simulink model "pha_0_9"  (R2023a)
settings: Solver=VariableStepAuto  StartTime=0.0  StopTime=100  RelTol=1e-3
libraries: fl_lib x55, SimscapeFluids_lib x25, nesl_utility x15, slpidlib x2, simulink x1
(part 2 of 2)

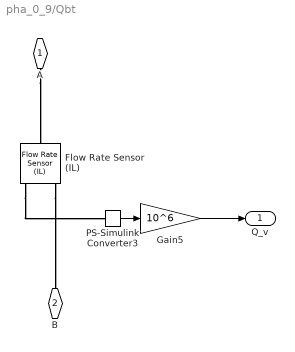
== system pha_0_9/Qbt ==
  Flow Rate Sensor (IL) : fl_lib/Isothermal Liquid/Sensors/Flow Rate Sensor (IL)  sensor_type=foundation.enum.mass_volumetric_sensor.mass_volumetric
      settings: InternalSimscapePortConfiguration="{\"Bottom\":[],\"Left\":[{\"id\":\"A\",\"label\":\"A\",\"type\":\"foundation.isothermal_liquid.isothermal_liquid\"}],\"Right\":[{\"id\":\"B\",\"label\":\"B\",\"type\":\"foundation.isothermal_liquid.isothermal_liquid\"},{\"id\":\"M\",\"label\":\"M\",\"type\":\"output\"},{\"id\":\"V\",\"label\":\"V\",\"type\":\"output\"}],\"Top\":[]}"
  Gain5 : Gain  Gain=10^6
  PS-Simulink Converter3 : nesl_utility/PS-Simulink Converter  PhysicalDomain=network_engine_domain  SubClassName=ps_output  LeftPortType=input  RightPortType=output  PseudoPeriodic=off  Frequencies=[]  VectorFormat=inherit  Unit=inherit  AffineConversion=off
  A : PMIOPort  Side=Left
  B : PMIOPort  Port=2  Side=Right
  Q_v : Outport
  wires:
  PS-Simulink Converter3/1 -> Gain5/1
  Gain5/1 -> Q_v/1
  connections:
  Flow Rate Sensor (IL)/RConn1 -- B/RConn1
  A/RConn1 -- Flow Rate Sensor (IL)/LConn1
  Flow Rate Sensor (IL)/RConn3 -- PS-Simulink Converter3/LConn1

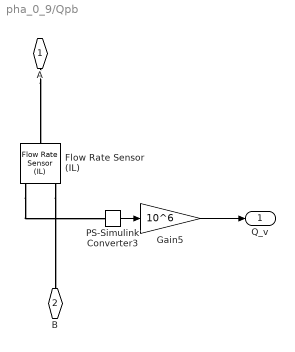
== system pha_0_9/Qpb ==
  Flow Rate Sensor (IL) : fl_lib/Isothermal Liquid/Sensors/Flow Rate Sensor (IL)  sensor_type=foundation.enum.mass_volumetric_sensor.mass_volumetric
      settings: InternalSimscapePortConfiguration="{\"Bottom\":[],\"Left\":[{\"id\":\"A\",\"label\":\"A\",\"type\":\"foundation.isothermal_liquid.isothermal_liquid\"}],\"Right\":[{\"id\":\"B\",\"label\":\"B\",\"type\":\"foundation.isothermal_liquid.isothermal_liquid\"},{\"id\":\"M\",\"label\":\"M\",\"type\":\"output\"},{\"id\":\"V\",\"label\":\"V\",\"type\":\"output\"}],\"Top\":[]}"
  Gain5 : Gain  Gain=10^6
  PS-Simulink Converter3 : nesl_utility/PS-Simulink Converter  PhysicalDomain=network_engine_domain  SubClassName=ps_output  LeftPortType=input  RightPortType=output  PseudoPeriodic=off  Frequencies=[]  VectorFormat=inherit  Unit=inherit  AffineConversion=off
  A : PMIOPort  Side=Left
  B : PMIOPort  Port=2  Side=Right
  Q_v : Outport
  wires:
  PS-Simulink Converter3/1 -> Gain5/1
  Gain5/1 -> Q_v/1
  connections:
  Flow Rate Sensor (IL)/RConn1 -- B/RConn1
  A/RConn1 -- Flow Rate Sensor (IL)/LConn1
  Flow Rate Sensor (IL)/RConn3 -- PS-Simulink Converter3/LConn1

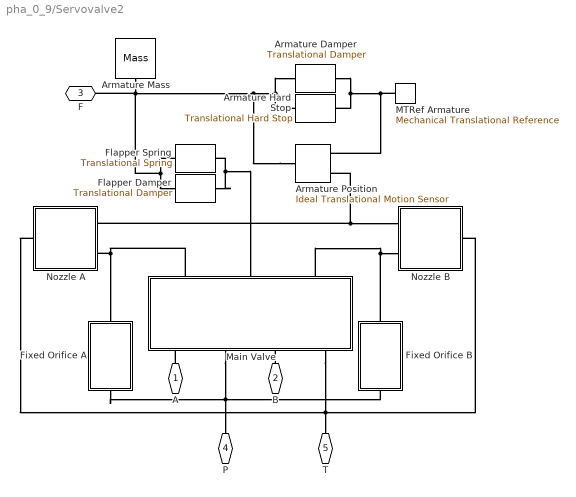
== system pha_0_9/Servovalve2 ==
  Armature Mass : fl_lib/Mechanical/Translational Elements/Mass  Tag=Factory Generic  mass=0.035 kg  num_ports=foundation.enum.numPorts2.one  v_specify=on  v_priority=High  v=0 m/s  v_nominal_specify=off  v_nominal_unit=m/s  v_nominal_value=1  f_specify=off  f_priority=High  f=0 N  f_nominal_specify=off  f_nominal_unit=N  f_nominal_value=1
  Armature Position : fl_lib/Mechanical/Mechanical Sensors/Ideal Translational Motion Sensor  Tag=Factory Generic  reference=foundation.enum.MeasurementReference.difference  acceleration_port=false  velocity_port=true  position_port=true  offset=0 m
  Armature Damper : fl_lib/Mechanical/Translational Elements/Translational Damper  Tag=Factory Generic  D=12.5 N/(m/s)  v_specify=off  v_priority=High  v=0 m/s  v_nominal_specify=off  v_nominal_unit=m/s  v_nominal_value=1  f_specify=off  f_priority=High  f=0 N  f_nominal_specify=off  f_nominal_unit=N  f_nominal_value=1
  Armature Hard Stop : fl_lib/Mechanical/Translational Elements/Translational Hard Stop  Tag=Factory Generic  upper_bnd=0.5 mm  lower_bnd=-0.5 mm  model=3  stiff_up=1e+06 N/m  stiff_low=1e+06 N/m  D_up=150 N/(m/s)  D_low=150 N/(m/s)  transition=0.1 mm  coeff_rest=0.7  v_tol=0.001 m/s  f_tol=0.001 N  x_specify=on  x_priority=High  x=0 m  x_nominal_specify=off  x_nominal_unit=m  x_nominal_value=1  v_specify=off  v_priority=High  v=0 m/s  v_nominal_specify=off  v_nominal_unit=m/s  v_nominal_value=1  f_specify=off  f_priority=High  f=0 N  f_nominal_specify=off  f_nominal_unit=N  f_nominal_value=1  M_specify=off  M_priority=None  M=0
  Fixed Orifice A : Subsystem
  Fixed Orifice B : Subsystem
  Flapper Damper : fl_lib/Mechanical/Translational Elements/Translational Damper  Tag=Factory Generic  D=51 N/(m/s)  v_specify=off  v_priority=High  v=0 m/s  v_nominal_specify=off  v_nominal_unit=m/s  v_nominal_value=1  f_specify=off  f_priority=High  f=0 N  f_nominal_specify=off  f_nominal_unit=N  f_nominal_value=1
  Flapper Spring : fl_lib/Mechanical/Translational Elements/Translational Spring  Tag=Factory Generic  spr_rate=1200 N/m  v_specify=off  v_priority=High  v=0 m/s  v_nominal_specify=off  v_nominal_unit=m/s  v_nominal_value=1  f_specify=off  f_priority=High  f=0 N  f_nominal_specify=off  f_nominal_unit=N  f_nominal_value=1  x_specify=on  x_priority=High  x=0 m  x_nominal_specify=off  x_nominal_unit=m  x_nominal_value=1
  MTRef Armature : fl_lib/Mechanical/Translational Elements/Mechanical Translational Reference  Tag=Factory Generic
  Main Valve : Subsystem  Tag=PublishSubsystem
  Nozzle A : Subsystem
  Nozzle B : Subsystem
  A : PMIOPort  Side=Left
  B : PMIOPort  Port=2  Side=Left
  F : PMIOPort  Port=3  Side=Right
  P : PMIOPort  Port=4  Side=Right
  T : PMIOPort  Port=5  Side=Right
  connections:
  Main Valve/RConn2 -- Fixed Orifice B/LConn1 -- Fixed Orifice A/LConn1 -- P/RConn1
  Armature Position/LConn1 -- Flapper Spring/LConn1 -- Flapper Damper/LConn1 -- F/RConn1 -- Armature Mass/LConn1 -- Armature Damper/LConn1 -- Armature Hard Stop/LConn1
  A/RConn1 -- Main Valve/RConn1
  B/RConn1 -- Main Valve/RConn3
  Flapper Damper/RConn1 -- Flapper Spring/RConn1 -- Main Valve/LConn2
  MTRef Armature/LConn1 -- Armature Position/RConn1 -- Armature Damper/RConn1 -- Armature Hard Stop/RConn1
  Main Valve/LConn1 -- Nozzle A/LConn2 -- Fixed Orifice A/RConn1
  Armature Position/RConn3 -- Nozzle B/LConn1 -- Nozzle A/LConn1
  Fixed Orifice B/RConn1 -- Main Valve/LConn3 -- Nozzle B/LConn2
  Nozzle A/RConn1 -- Nozzle B/RConn1 -- T/RConn1 -- Main Valve/RConn4

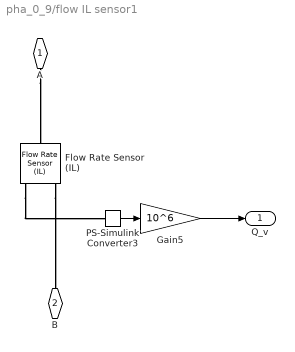
== system pha_0_9/flow IL sensor1 ==
  Flow Rate Sensor (IL) : fl_lib/Isothermal Liquid/Sensors/Flow Rate Sensor (IL)  sensor_type=foundation.enum.mass_volumetric_sensor.mass_volumetric
      settings: InternalSimscapePortConfiguration="{\"Bottom\":[],\"Left\":[{\"id\":\"A\",\"label\":\"A\",\"type\":\"foundation.isothermal_liquid.isothermal_liquid\"}],\"Right\":[{\"id\":\"B\",\"label\":\"B\",\"type\":\"foundation.isothermal_liquid.isothermal_liquid\"},{\"id\":\"M\",\"label\":\"M\",\"type\":\"output\"},{\"id\":\"V\",\"label\":\"V\",\"type\":\"output\"}],\"Top\":[]}"
  Gain5 : Gain  Gain=10^6
  PS-Simulink Converter3 : nesl_utility/PS-Simulink Converter  PhysicalDomain=network_engine_domain  SubClassName=ps_output  LeftPortType=input  RightPortType=output  PseudoPeriodic=off  Frequencies=[]  VectorFormat=inherit  Unit=inherit  AffineConversion=off
  A : PMIOPort  Side=Left
  B : PMIOPort  Port=2  Side=Right
  Q_v : Outport
  wires:
  PS-Simulink Converter3/1 -> Gain5/1
  Gain5/1 -> Q_v/1
  connections:
  Flow Rate Sensor (IL)/RConn1 -- B/RConn1
  A/RConn1 -- Flow Rate Sensor (IL)/LConn1
  Flow Rate Sensor (IL)/RConn3 -- PS-Simulink Converter3/LConn1

== system pha_0_9/flow sensor1 ==
  Flow Rate Sensor (TL)3 : fl_lib/Thermal Liquid/Sensors/Flow Rate Sensor (TL)  mass_flow_measure=true  volumetric_flow_measure=true  energy_flow_measure=true
      settings: InternalSimscapePortConfiguration="{\"Bottom\":[{\"id\":\"PHI\",\"label\":\"φ\",\"type\":\"output\"}],\"Left\":[{\"id\":\"A\",\"label\":\"A\",\"type\":\"foundation.thermal_liquid.thermal_liquid\"}],\"Right\":[{\"id\":\"B\",\"label\":\"B\",\"type\":\"foundation.thermal_liquid.thermal_liquid\"},{\"id\":\"M\",\"label\":\"M\",\"type\":\"output\"},{\"id\":\"V\",\"label\":\"V\",\"type\":\"output\"}],\"Top\":[]}"
  Gain5 : Gain  Gain=10^6
  PS-Simulink Converter3 : nesl_utility/PS-Simulink Converter  PhysicalDomain=network_engine_domain  SubClassName=ps_output  LeftPortType=input  RightPortType=output  PseudoPeriodic=off  Frequencies=[]  VectorFormat=inherit  Unit=inherit  AffineConversion=off
  A : PMIOPort  Side=Left
  B : PMIOPort  Port=2  Side=Right
  Q_v : Outport
  wires:
  PS-Simulink Converter3/1 -> Gain5/1
  Gain5/1 -> Q_v/1
  connections:
  PS-Simulink Converter3/LConn1 -- Flow Rate Sensor (TL)3/RConn3
  Flow Rate Sensor (TL)3/RConn1 -- B/RConn1
  A/RConn1 -- Flow Rate Sensor (TL)3/LConn1

== system pha_0_9/flow sensor2 ==
  Flow Rate Sensor (TL)3 : fl_lib/Thermal Liquid/Sensors/Flow Rate Sensor (TL)  mass_flow_measure=true  volumetric_flow_measure=true  energy_flow_measure=true
      settings: InternalSimscapePortConfiguration="{\"Bottom\":[{\"id\":\"PHI\",\"label\":\"φ\",\"type\":\"output\"}],\"Left\":[{\"id\":\"A\",\"label\":\"A\",\"type\":\"foundation.thermal_liquid.thermal_liquid\"}],\"Right\":[{\"id\":\"B\",\"label\":\"B\",\"type\":\"foundation.thermal_liquid.thermal_liquid\"},{\"id\":\"M\",\"label\":\"M\",\"type\":\"output\"},{\"id\":\"V\",\"label\":\"V\",\"type\":\"output\"}],\"Top\":[]}"
  Gain5 : Gain  Gain=10^6
  PS-Simulink Converter3 : nesl_utility/PS-Simulink Converter  PhysicalDomain=network_engine_domain  SubClassName=ps_output  LeftPortType=input  RightPortType=output  PseudoPeriodic=off  Frequencies=[]  VectorFormat=inherit  Unit=inherit  AffineConversion=off
  A : PMIOPort  Side=Left
  B : PMIOPort  Port=2  Side=Right
  Q_v : Outport
  wires:
  PS-Simulink Converter3/1 -> Gain5/1
  Gain5/1 -> Q_v/1
  connections:
  PS-Simulink Converter3/LConn1 -- Flow Rate Sensor (TL)3/RConn3
  Flow Rate Sensor (TL)3/RConn1 -- B/RConn1
  A/RConn1 -- Flow Rate Sensor (TL)3/LConn1

== system pha_0_9/flow sensor3 ==
  Flow Rate Sensor (TL)3 : fl_lib/Thermal Liquid/Sensors/Flow Rate Sensor (TL)  mass_flow_measure=true  volumetric_flow_measure=true  energy_flow_measure=true
      settings: InternalSimscapePortConfiguration="{\"Bottom\":[{\"id\":\"PHI\",\"label\":\"φ\",\"type\":\"output\"}],\"Left\":[{\"id\":\"A\",\"label\":\"A\",\"type\":\"foundation.thermal_liquid.thermal_liquid\"}],\"Right\":[{\"id\":\"B\",\"label\":\"B\",\"type\":\"foundation.thermal_liquid.thermal_liquid\"},{\"id\":\"M\",\"label\":\"M\",\"type\":\"output\"},{\"id\":\"V\",\"label\":\"V\",\"type\":\"output\"}],\"Top\":[]}"
  Gain5 : Gain  Gain=10^6
  PS-Simulink Converter3 : nesl_utility/PS-Simulink Converter  PhysicalDomain=network_engine_domain  SubClassName=ps_output  LeftPortType=input  RightPortType=output  PseudoPeriodic=off  Frequencies=[]  VectorFormat=inherit  Unit=inherit  AffineConversion=off
  A : PMIOPort  Side=Left
  B : PMIOPort  Port=2  Side=Right
  Q_v : Outport
  wires:
  PS-Simulink Converter3/1 -> Gain5/1
  Gain5/1 -> Q_v/1
  connections:
  PS-Simulink Converter3/LConn1 -- Flow Rate Sensor (TL)3/RConn3
  Flow Rate Sensor (TL)3/RConn1 -- B/RConn1
  A/RConn1 -- Flow Rate Sensor (TL)3/LConn1

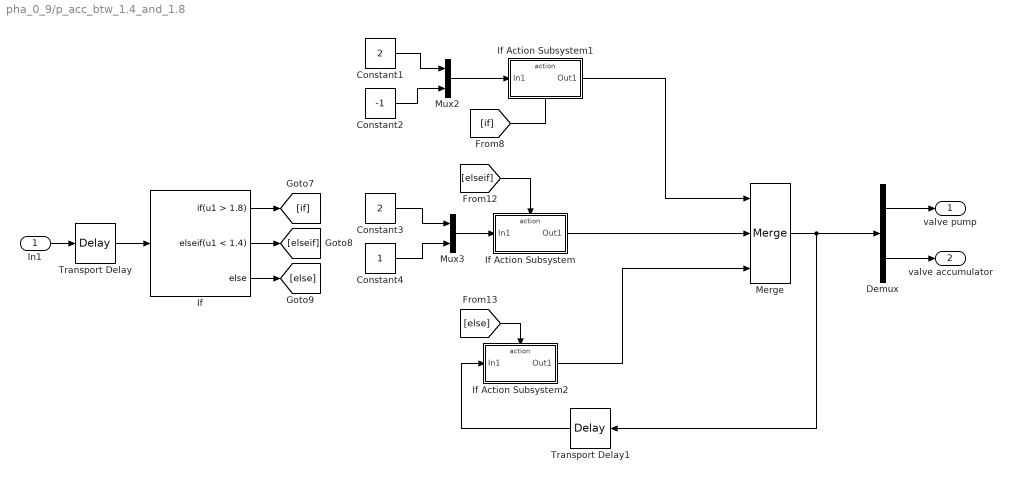
== system pha_0_9/p_acc_btw_1.4_and_1.8 ==
  In1 : Inport
  Constant1 : Constant  Value=2
  Constant2 : Constant  Value=-1
  Constant3 : Constant  Value=2
  Constant4 : Constant
  Demux : Demux  Outputs=2
  If : If  IfExpression=u1 > 1.8  ElseIfExpressions=u1 < 1.4
  If Action Subsystem : Subsystem  TreatAsAtomicUnit=on
  If Action Subsystem1 : Subsystem  TreatAsAtomicUnit=on
  If Action Subsystem2 : Subsystem  TreatAsAtomicUnit=on
  Merge : Merge  Inputs=3
  Mux2 : Mux  Inputs=2
  Mux3 : Mux  Inputs=2
  Transport Delay : TransportDelay  DelayTime=0.001
  Transport Delay1 : TransportDelay  DelayTime=0.001
  valve pump : Outport
  valve accumulator : Outport  Port=2
  wires:
  If/3 -> [else]
  [else] -> If Action Subsystem2/Action
  Merge/1 -> Transport Delay1/1, Demux/1
  Constant3/1 -> Mux3/1
  If/2 -> [elseif]
  Transport Delay1/1 -> If Action Subsystem2/1(In1)
  Constant1/1 -> Mux2/1
  Demux/1 -> valve pump/1
  Constant2/1 -> Mux2/2
  Mux3/1 -> If Action Subsystem/1(In1)
  Constant4/1 -> Mux3/2
  Transport Delay/1 -> If/1
  [elseif] -> If Action Subsystem/Action
  If/1 -> [if]
  Demux/2 -> valve accumulator/1
  In1/1 -> Transport Delay/1
  If Action Subsystem/1(Out1) -> Merge/2
  If Action Subsystem2/1(Out1) -> Merge/3
  If Action Subsystem1/1(Out1) -> Merge/1
  Mux2/1 -> If Action Subsystem1/1(In1)
  [if] -> If Action Subsystem1/Action

== system pha_0_9/pressure sensor ==
  Gain : Gain  Gain=10^(-5)
  PS-Simulink Converter1 : nesl_utility/PS-Simulink Converter  PhysicalDomain=network_engine_domain  SubClassName=ps_output  LeftPortType=input  RightPortType=output  PseudoPeriodic=off  Frequencies=[]  VectorFormat=inherit  Unit=inherit  AffineConversion=off
  Pressure & Temperature Sensor (TL) : fl_lib/Thermal Liquid/Sensors/Pressure & Temperature Sensor (TL)  reference=foundation.enum.MeasurementReference.absolute  pressure=true  pressure_spec=foundation.enum.PressureMeasementSpec.Absolute  temperature=false
      settings: InternalSimscapePortConfiguration="{\"Bottom\":[],\"Left\":[{\"id\":\"A\",\"label\":\"A\",\"type\":\"foundation.thermal_liquid.thermal_liquid\"}],\"Right\":[{\"id\":\"Pa\",\"label\":\"Pa\",\"type\":\"output\"}],\"Top\":[]}"
  A : PMIOPort  Side=Left
  bar : Outport
  wires:
  PS-Simulink Converter1/1 -> Gain/1
  Gain/1 -> bar/1
  connections:
  PS-Simulink Converter1/LConn1 -- Pressure & Temperature Sensor (TL)/RConn1
  Pressure & Temperature Sensor (TL)/LConn1 -- A/RConn1

== system pha_0_9/pressure sensor1 ==
  Gain : Gain  Gain=10^(-5)
  PS-Simulink Converter1 : nesl_utility/PS-Simulink Converter  PhysicalDomain=network_engine_domain  SubClassName=ps_output  LeftPortType=input  RightPortType=output  PseudoPeriodic=off  Frequencies=[]  VectorFormat=inherit  Unit=inherit  AffineConversion=off
  Pressure & Temperature Sensor (TL) : fl_lib/Thermal Liquid/Sensors/Pressure & Temperature Sensor (TL)  reference=foundation.enum.MeasurementReference.absolute  pressure=true  pressure_spec=foundation.enum.PressureMeasementSpec.Absolute  temperature=false
      settings: InternalSimscapePortConfiguration="{\"Bottom\":[],\"Left\":[{\"id\":\"A\",\"label\":\"A\",\"type\":\"foundation.thermal_liquid.thermal_liquid\"}],\"Right\":[{\"id\":\"Pa\",\"label\":\"Pa\",\"type\":\"output\"}],\"Top\":[]}"
  A : PMIOPort  Side=Left
  bar : Outport
  wires:
  PS-Simulink Converter1/1 -> Gain/1
  Gain/1 -> bar/1
  connections:
  PS-Simulink Converter1/LConn1 -- Pressure & Temperature Sensor (TL)/RConn1
  Pressure & Temperature Sensor (TL)/LConn1 -- A/RConn1

== system pha_0_9/pressure sensor2 ==
  Gain : Gain  Gain=10^(-5)
  PS-Simulink Converter1 : nesl_utility/PS-Simulink Converter  PhysicalDomain=network_engine_domain  SubClassName=ps_output  LeftPortType=input  RightPortType=output  PseudoPeriodic=off  Frequencies=[]  VectorFormat=inherit  Unit=inherit  AffineConversion=off
  Pressure & Temperature Sensor (TL) : fl_lib/Thermal Liquid/Sensors/Pressure & Temperature Sensor (TL)  reference=foundation.enum.MeasurementReference.absolute  pressure=true  pressure_spec=foundation.enum.PressureMeasementSpec.Absolute  temperature=false
      settings: InternalSimscapePortConfiguration="{\"Bottom\":[],\"Left\":[{\"id\":\"A\",\"label\":\"A\",\"type\":\"foundation.thermal_liquid.thermal_liquid\"}],\"Right\":[{\"id\":\"Pa\",\"label\":\"Pa\",\"type\":\"output\"}],\"Top\":[]}"
  A : PMIOPort  Side=Left
  bar : Outport
  wires:
  PS-Simulink Converter1/1 -> Gain/1
  Gain/1 -> bar/1
  connections:
  PS-Simulink Converter1/LConn1 -- Pressure & Temperature Sensor (TL)/RConn1
  Pressure & Temperature Sensor (TL)/LConn1 -- A/RConn1

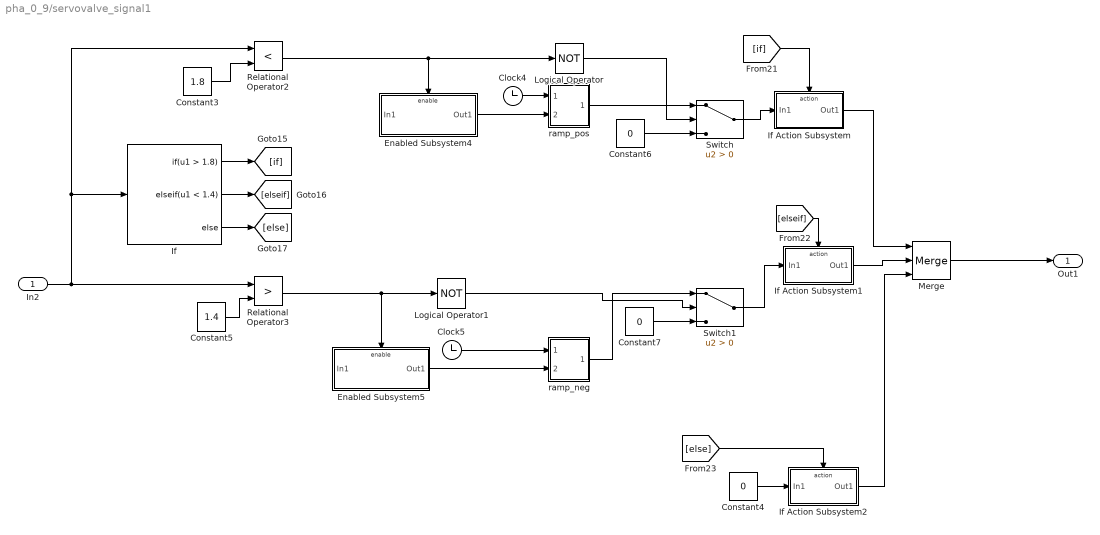
== system pha_0_9/servovalve_signal1 ==
  In2 : Inport
  Clock4 : Clock
  Clock5 : Clock
  Constant3 : Constant  Value=1.8
  Constant4 : Constant  Value=0
  Constant5 : Constant  Value=1.4
  Constant6 : Constant  Value=0
  Constant7 : Constant  Value=0
  Enabled Subsystem4 : Subsystem  TreatAsAtomicUnit=on
  Enabled Subsystem5 : Subsystem  TreatAsAtomicUnit=on
  If : If  IfExpression=u1 > 1.8  ElseIfExpressions=u1 < 1.4
  If Action Subsystem : Subsystem  TreatAsAtomicUnit=on
  If Action Subsystem1 : Subsystem  TreatAsAtomicUnit=on
  If Action Subsystem2 : Subsystem  TreatAsAtomicUnit=on
  Logical Operator : Logic  Operator=NOT  AllPortsSameDT=off  OutDataTypeStr=boolean
  Logical Operator1 : Logic  Operator=NOT  AllPortsSameDT=off  OutDataTypeStr=boolean
  Merge : Merge  Inputs=3
  Relational Operator2 : RelationalOperator  Operator=<  OutDataTypeStr=boolean  RndMeth=Simplest  InputSameDT=off
  Relational Operator3 : RelationalOperator  Operator=>  OutDataTypeStr=boolean  RndMeth=Simplest  InputSameDT=off
  Switch : Switch  Criteria=u2 > Threshold  SaturateOnIntegerOverflow=off  InputSameDT=off
  Switch1 : Switch  Criteria=u2 > Threshold  SaturateOnIntegerOverflow=off  InputSameDT=off
  ramp_neg : Subsystem
  ramp_pos : Subsystem
  Out1 : Outport
  wires:
  Relational Operator2/1 -> Logical Operator/1, Enabled Subsystem4/Enable
  Enabled Subsystem4/1(Out1) -> ramp_pos/2(In2)
  [if] -> If Action Subsystem/Action
  [else] -> If Action Subsystem2/Action
  Relational Operator3/1 -> Logical Operator1/1, Enabled Subsystem5/Enable
  If Action Subsystem1/1(Out1) -> Merge/2
  ramp_neg/1(Out1) -> Switch1/1
  Switch1/1 -> If Action Subsystem1/1(In1)
  In2/1 -> If/1, Relational Operator2/1, Relational Operator3/1
  Merge/1 -> Out1/1
  Logical Operator1/1 -> Switch1/2
  Clock4/1 -> ramp_pos/1(In1)
  Enabled Subsystem5/1(Out1) -> ramp_neg/2(In2)
  Constant4/1 -> If Action Subsystem2/1(In1)
  Switch/1 -> If Action Subsystem/1(In1)
  [elseif] -> If Action Subsystem1/Action
  If Action Subsystem/1(Out1) -> Merge/1
  Constant7/1 -> Switch1/3
  If/2 -> [elseif]
  Constant3/1 -> Relational Operator2/2
  If/1 -> [if]
  Constant6/1 -> Switch/3
  Constant5/1 -> Relational Operator3/2
  Clock5/1 -> ramp_neg/1(In1)
  If Action Subsystem2/1(Out1) -> Merge/3
  Logical Operator/1 -> Switch/2
  If/3 -> [else]
  ramp_pos/1(Out1) -> Switch/1

== system pha_0_9/Servovalve2/Fixed Orifice A ==
  Fixed Orifice A : SimscapeFluids_lib/Isothermal Liquid/Valves & Orifices/Orifices/Orifice (IL)  Tag=Factory Generic  orifice_type=1  constant_orifice_spec=fluids.isothermal_liquid.valves_orifices.orifices.enum.constant_orifice_spec.area  variable_orifice_spec=fluids.isothermal_liquid.valves_orifices.orifices.enum.orifice_spec.linear  orifice_area_constant=2 mm^2  p_diff_TLU_constant=[-4, -3, -2, -1, -.5, 0, .5, 1, 2, 3, 4] MPa  vol_flow_TLU_constant=[-2.44, -2.12, -1.68, -1.22, -.84, 0, .85, 1.21, 1.7, 2.09, 2.41] .* 1e-3 m^3/s  S_min=0 m  del_S=5e-3 m  open_orientation=fluids.isothermal_liquid.valves_orifices.orifices.enum.orifice_orientation.positive  area_max=1e-4 m^2  area_leak=1e-10 m^2  S_TLU=[0, .002, .004, .007, .017] m  orifice_area_TLU=[1e-09, 2.0352e-07, 4.0736e-05, .00011438, .00034356] m^2  area=inf mm^2  Cd=0.7  Re_c=150  smoothing_factor=0.01  pressure_recovery=false  S_vol_flow_TLU=[0, .002, .004, .007, .017] m  p_diff_TLU=[.3, .5, .7] MPa  vol_flow_TLU=1e-3 * [1.7e-05, 2e-05, 2.6e-05; .0035, .0045, .0053; .7, .9, 1.06; 1.96, 2.5, 3; 6, 7.7, 9.13] m^3/s  enable_faults=simscape.enum.onoff.off  fault_action=fluids.enum.FaultOpening.Closed  external_fault=fluids.enum.FaultExternalTrigger.Off  temporal_fault=simscape.enum.onoff.off  fault_time=5 s  report_fault=simscape.enum.assert.action.none
      settings: InternalSimscapePortConfiguration="{\"Bottom\":[],\"Left\":[{\"id\":\"A\",\"label\":\"A\",\"type\":\"foundation.isothermal_liquid.isothermal_liquid\"}],\"Right\":[{\"id\":\"B\",\"label\":\"B\",\"type\":\"foundation.isothermal_liquid.isothermal_liquid\"}],\"Top\":[]}"
  B : PMIOPort  Side=Right
  A : PMIOPort  Port=2  Side=Left
  connections:
  A/RConn1 -- Fixed Orifice A/LConn1
  B/RConn1 -- Fixed Orifice A/RConn1

== system pha_0_9/Servovalve2/Fixed Orifice B ==
  Fixed Orifice B : SimscapeFluids_lib/Isothermal Liquid/Valves & Orifices/Orifices/Orifice (IL)  Tag=Factory Generic  orifice_type=1  constant_orifice_spec=fluids.isothermal_liquid.valves_orifices.orifices.enum.constant_orifice_spec.area  variable_orifice_spec=fluids.isothermal_liquid.valves_orifices.orifices.enum.orifice_spec.linear  orifice_area_constant=2 mm^2  p_diff_TLU_constant=[-4, -3, -2, -1, -.5, 0, .5, 1, 2, 3, 4] MPa  vol_flow_TLU_constant=[-2.44, -2.12, -1.68, -1.22, -.84, 0, .85, 1.21, 1.7, 2.09, 2.41] .* 1e-3 m^3/s  S_min=0 m  del_S=5e-3 m  open_orientation=fluids.isothermal_liquid.valves_orifices.orifices.enum.orifice_orientation.positive  area_max=1e-4 m^2  area_leak=1e-10 m^2  S_TLU=[0, .002, .004, .007, .017] m  orifice_area_TLU=[1e-09, 2.0352e-07, 4.0736e-05, .00011438, .00034356] m^2  area=inf mm^2  Cd=0.7  Re_c=150  smoothing_factor=0.01  pressure_recovery=false  S_vol_flow_TLU=[0, .002, .004, .007, .017] m  p_diff_TLU=[.3, .5, .7] MPa  vol_flow_TLU=1e-3 * [1.7e-05, 2e-05, 2.6e-05; .0035, .0045, .0053; .7, .9, 1.06; 1.96, 2.5, 3; 6, 7.7, 9.13] m^3/s  enable_faults=simscape.enum.onoff.off  fault_action=fluids.enum.FaultOpening.Closed  external_fault=fluids.enum.FaultExternalTrigger.Off  temporal_fault=simscape.enum.onoff.off  fault_time=5 s  report_fault=simscape.enum.assert.action.none
      settings: InternalSimscapePortConfiguration="{\"Bottom\":[],\"Left\":[{\"id\":\"A\",\"label\":\"A\",\"type\":\"foundation.isothermal_liquid.isothermal_liquid\"}],\"Right\":[{\"id\":\"B\",\"label\":\"B\",\"type\":\"foundation.isothermal_liquid.isothermal_liquid\"}],\"Top\":[]}"
  B : PMIOPort  Side=Right
  A : PMIOPort  Port=2  Side=Left
  connections:
  A/RConn1 -- Fixed Orifice B/LConn1
  B/RConn1 -- Fixed Orifice B/RConn1

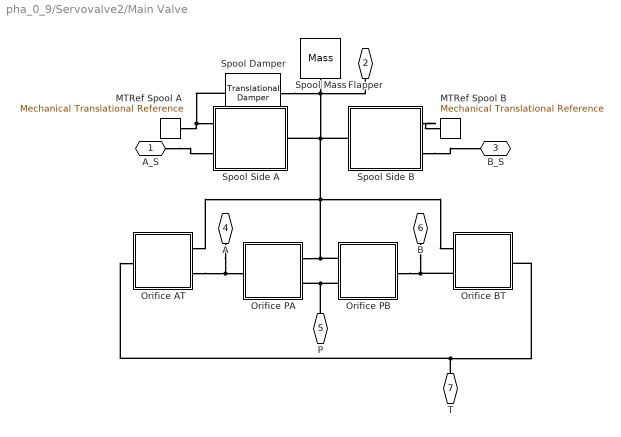
== system pha_0_9/Servovalve2/Main Valve ==
  MTRef Spool A : fl_lib/Mechanical/Translational Elements/Mechanical Translational Reference  Tag=Factory Generic
  MTRef Spool B : fl_lib/Mechanical/Translational Elements/Mechanical Translational Reference  Tag=Factory Generic
  Orifice AT : Subsystem  Tag=PublishSubsystem
  Orifice BT : Subsystem
  Orifice PA : Subsystem
  Orifice PB : Subsystem
  Spool Damper : fl_lib/Mechanical/Translational Elements/Translational Damper  Tag=Factory Generic  D=362 N/(m/s)  v_specify=off  v_priority=High  v=0 m/s  v_nominal_specify=off  v_nominal_unit=m/s  v_nominal_value=1  f_specify=off  f_priority=High  f=0 N  f_nominal_specify=off  f_nominal_unit=N  f_nominal_value=1
  Spool Mass : fl_lib/Mechanical/Translational Elements/Mass  Tag=Factory Generic  mass=0.124 kg  num_ports=foundation.enum.numPorts2.one  v_specify=on  v_priority=High  v=0 m/s  v_nominal_specify=off  v_nominal_unit=m/s  v_nominal_value=1  f_specify=off  f_priority=High  f=0 N  f_nominal_specify=off  f_nominal_unit=N  f_nominal_value=1
  Spool Side A : Subsystem
  Spool Side B : Subsystem
  A_S : PMIOPort  Side=Left
  Flapper : PMIOPort  Port=2  Side=Left
  B_S : PMIOPort  Port=3  Side=Left
  A : PMIOPort  Port=4  Side=Right
  P : PMIOPort  Port=5  Side=Right
  B : PMIOPort  Port=6  Side=Right
  T : PMIOPort  Port=7  Side=Right
  connections:
  A/RConn1 -- Orifice AT/LConn2 -- Orifice PA/RConn1
  P/RConn1 -- Orifice PB/LConn2 -- Orifice PA/LConn2
  Orifice BT/LConn2 -- Orifice PB/RConn1 -- B/RConn1
  T/RConn1 -- Orifice AT/RConn1 -- Orifice BT/RConn1
  MTRef Spool A/LConn1 -- Spool Damper/RConn1 -- Spool Side A/LConn1
  A_S/RConn1 -- Spool Side A/LConn2
  Orifice PA/LConn1 -- Orifice PB/LConn1 -- Orifice BT/LConn1 -- Orifice AT/LConn1 -- Spool Side B/RConn1 -- Spool Side A/RConn1 -- Spool Damper/LConn1 -- Spool Mass/LConn1 -- Flapper/RConn1
  Spool Side B/LConn1 -- MTRef Spool B/LConn1
  Spool Side B/LConn2 -- B_S/RConn1

== system pha_0_9/Servovalve2/Nozzle A ==
  Nozzle A : SimscapeFluids_lib/Isothermal Liquid/Valves & Orifices/Orifices/Orifice (IL)  Tag=Factory Generic  orifice_type=foundation.enum.constant_variable.variable  constant_orifice_spec=fluids.isothermal_liquid.valves_orifices.orifices.enum.constant_orifice_spec.area  variable_orifice_spec=1  orifice_area_constant=1e-3 m^2  p_diff_TLU_constant=[-4, -3, -2, -1, -.5, 0, .5, 1, 2, 3, 4] MPa  vol_flow_TLU_constant=[-2.44, -2.12, -1.68, -1.22, -.84, 0, .85, 1.21, 1.7, 2.09, 2.41] .* 1e-3 m^3/s  S_min=-2.9981e-07 m^2/mm  del_S=5.9981e-07 m^2/mm  open_orientation=1  area_max=3.14 mm^2  area_leak=1e-9 m^2  S_TLU="[  -0.002 0 0.005 0.015 ] - 0.001*(0.3) m"  orifice_area_TLU="[  1e-12 4e-12 1e-05 1.02e-05 ] m^2"  area=inf m^2  Cd=0.7  Re_c=150  smoothing_factor=0  pressure_recovery=false  S_vol_flow_TLU="[  -0.002 0 0.005 0.015 ] - 0.001*(0.3) m"  p_diff_TLU="[  -5e+06 -2e+06 2e+06 5e+06 ] Pa"  vol_flow_TLU="[  -1e-12 -6e-14 6e+12 1e+11 ; -8e-08 -4e-08 4e+06 8e+06 ; -0.0025 -0.00103 0.001 0.0024 ; -0.00258 -0.001032 0.00106 0.00247 ; ] m^3/s"  enable_faults=simscape.enum.onoff.off  fault_action=fluids.enum.FaultOpening.Closed  external_fault=fluids.enum.FaultExternalTrigger.Off  temporal_fault=simscape.enum.onoff.off  fault_time=5 s  report_fault=simscape.enum.assert.action.none
      settings: InternalSimscapePortConfiguration="{\"Bottom\":[],\"Left\":[{\"id\":\"A\",\"label\":\"A\",\"type\":\"foundation.isothermal_liquid.isothermal_liquid\"},{\"id\":\"S\",\"label\":\"S\",\"type\":\"input\"}],\"Right\":[{\"id\":\"B\",\"label\":\"B\",\"type\":\"foundation.isothermal_liquid.isothermal_liquid\"}],\"Top\":[]}"
  S : PMIOPort  Side=Left
  A : PMIOPort  Port=2  Side=Left
  B : PMIOPort  Port=3  Side=Right
  connections:
  Nozzle A/LConn1 -- A/RConn1
  Nozzle A/LConn2 -- S/RConn1
  B/RConn1 -- Nozzle A/RConn1

== system pha_0_9/Servovalve2/Nozzle B ==
  Nozzle B : SimscapeFluids_lib/Isothermal Liquid/Valves & Orifices/Orifices/Orifice (IL)  Tag=Factory Generic  orifice_type=foundation.enum.constant_variable.variable  constant_orifice_spec=fluids.isothermal_liquid.valves_orifices.orifices.enum.constant_orifice_spec.area  variable_orifice_spec=1  orifice_area_constant=1e-3 m^2  p_diff_TLU_constant=[-4, -3, -2, -1, -.5, 0, .5, 1, 2, 3, 4] MPa  vol_flow_TLU_constant=[-2.44, -2.12, -1.68, -1.22, -.84, 0, .85, 1.21, 1.7, 2.09, 2.41] .* 1e-3 m^3/s  S_min=2.9981e-07 m^2/mm  del_S=5.9981e-07 m^2/mm  open_orientation=-1  area_max=3.14 mm^2  area_leak=1e-9 m^2  S_TLU="-([  -0.002 0 0.005 0.015 ]) + 0.001*(0.3) m"  orifice_area_TLU="[  1e-12 4e-12 1e-05 1.02e-05 ] m^2"  area=inf m^2  Cd=0.7  Re_c=150  smoothing_factor=0  pressure_recovery=false  S_vol_flow_TLU="-([  -0.002 0 0.005 0.015 ]) + 0.001*(0.3) m"  p_diff_TLU="[  -5e+06 -2e+06 2e+06 5e+06 ] Pa"  vol_flow_TLU="[  -1e-12 -6e-14 6e+12 1e+11 ; -8e-08 -4e-08 4e+06 8e+06 ; -0.0025 -0.00103 0.001 0.0024 ; -0.00258 -0.001032 0.00106 0.00247 ; ] m^3/s"  enable_faults=simscape.enum.onoff.off  fault_action=fluids.enum.FaultOpening.Closed  external_fault=fluids.enum.FaultExternalTrigger.Off  temporal_fault=simscape.enum.onoff.off  fault_time=5 s  report_fault=simscape.enum.assert.action.none
      settings: InternalSimscapePortConfiguration="{\"Bottom\":[],\"Left\":[{\"id\":\"A\",\"label\":\"A\",\"type\":\"foundation.isothermal_liquid.isothermal_liquid\"},{\"id\":\"S\",\"label\":\"S\",\"type\":\"input\"}],\"Right\":[{\"id\":\"B\",\"label\":\"B\",\"type\":\"foundation.isothermal_liquid.isothermal_liquid\"}],\"Top\":[]}"
  S : PMIOPort  Side=Left
  A : PMIOPort  Port=2  Side=Left
  B : PMIOPort  Port=3  Side=Right
  connections:
  A/RConn1 -- Nozzle B/LConn1
  S/RConn1 -- Nozzle B/LConn2
  B/RConn1 -- Nozzle B/RConn1

== system pha_0_9/p_acc_btw_1.4_and_1.8/If Action Subsystem ==
  In1 : Inport
  Action Port : ActionPort  ActionPortLabel=elseif(u1 < 1.4)
  Out1 : Outport  InitialOutput=[0 0]
  wires:
  In1/1 -> Out1/1

== system pha_0_9/p_acc_btw_1.4_and_1.8/If Action Subsystem1 ==
  In1 : Inport
  Action Port : ActionPort  ActionPortLabel=if(u1 > 1.8)
  Out1 : Outport
  wires:
  In1/1 -> Out1/1

== system pha_0_9/p_acc_btw_1.4_and_1.8/If Action Subsystem2 ==
  In1 : Inport
  Action Port : ActionPort  ActionPortLabel=else
  Out1 : Outport  InitialOutput=[0 0]
  wires:
  In1/1 -> Out1/1

== system pha_0_9/servovalve_signal1/Enabled Subsystem4 ==
  In1 : Inport
  Enable : EnablePort
  Clock : Clock
  Out1 : Outport
  wires:
  Clock/1 -> Out1/1

== system pha_0_9/servovalve_signal1/Enabled Subsystem5 ==
  In1 : Inport
  Enable : EnablePort
  Clock : Clock
  Out1 : Outport
  wires:
  Clock/1 -> Out1/1

== system pha_0_9/servovalve_signal1/If Action Subsystem ==
  In1 : Inport
  Action Port : ActionPort
  Out1 : Outport
  wires:
  In1/1 -> Out1/1

== system pha_0_9/servovalve_signal1/If Action Subsystem1 ==
  In1 : Inport
  Action Port : ActionPort
  Out1 : Outport
  wires:
  In1/1 -> Out1/1

== system pha_0_9/servovalve_signal1/If Action Subsystem2 ==
  In1 : Inport
  Action Port : ActionPort
  Out1 : Outport
  wires:
  In1/1 -> Out1/1

== system pha_0_9/servovalve_signal1/ramp_neg ==
  In1 : Inport
  In2 : Inport  Port=2
  Gain6 : Gain
  Subtract5 : Sum  Inputs=+-
  Out1 : Outport
  wires:
  Subtract5/1 -> Gain6/1
  In1/1 -> Subtract5/1
  Gain6/1 -> Out1/1
  In2/1 -> Subtract5/2

== system pha_0_9/servovalve_signal1/ramp_pos ==
  In1 : Inport
  In2 : Inport  Port=2
  Gain4 : Gain  Gain=-1
  Subtract4 : Sum  Inputs=+-
  Out1 : Outport
  wires:
  Subtract4/1 -> Gain4/1
  Gain4/1 -> Out1/1
  In1/1 -> Subtract4/1
  In2/1 -> Subtract4/2

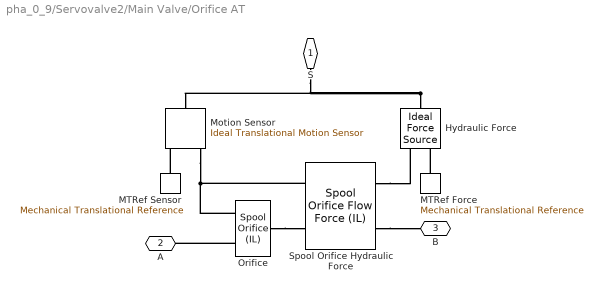
== system pha_0_9/Servovalve2/Main Valve/Orifice AT ==
  Hydraulic Force : fl_lib/Mechanical/Mechanical Sources/Ideal Force Source  Tag=Factory Generic
  MTRef Force : fl_lib/Mechanical/Translational Elements/Mechanical Translational Reference  Tag=Factory Generic
  MTRef Sensor : fl_lib/Mechanical/Translational Elements/Mechanical Translational Reference  Tag=Factory Generic
  Motion Sensor : fl_lib/Mechanical/Mechanical Sensors/Ideal Translational Motion Sensor  Tag=Factory Generic  reference=foundation.enum.MeasurementReference.difference  acceleration_port=false  velocity_port=true  position_port=true  offset=0 m
  Orifice : SimscapeFluids_lib/Isothermal Liquid/Valves & Orifices/Orifices/Spool Orifice (IL)  Tag=Factory Generic  orifice_spec=2  diameter_hole=5e-3 m  num_hole=6  width=24.5 mm  del_S_max=1 m  S_min=0.01 mm  open_orientation=-1  flow_force_spec=false  clearance=1e-5 m  area_leak=1e-9 m^2  area=inf m^2  Cd=0.7  Re_c=150  smoothing_factor=0  pressure_recovery=false
      settings: InternalSimscapePortConfiguration="{\"Bottom\":[],\"Left\":[{\"id\":\"S\",\"label\":\"S\",\"type\":\"input\"},{\"id\":\"A\",\"label\":\"A\",\"type\":\"foundation.isothermal_liquid.isothermal_liquid\"}],\"Right\":[{\"id\":\"B\",\"label\":\"B\",\"type\":\"foundation.isothermal_liquid.isothermal_liquid\"}],\"Top\":[]}"
  Spool Orifice Hydraulic Force : SimscapeFluids_lib/Isothermal Liquid/Valves & Orifices/Valve Actuators & Forces/Spool Orifice Flow Force (IL)  orifice_spec=2  diameter_hole=0.005 m  num_hole=4  width=24.5 mm  del_S_max=1 m  S_min=0.01 mm  open_orientation=-1  clearance=0.05 mm  area_leak=(24.5)*(0.05) mm^2  smoothing_factor=0
      settings: LibrarySourceBlock=SimscapeFluids_lib/Isothermal Liquid/Valves & Orifices/Valve Actuators & Forces/Spool Orifice Flow Force (IL)  InternalSimscapePortConfiguration="{\"Bottom\":[],\"Left\":[{\"id\":\"A\",\"label\":\"A\",\"type\":\"foundation.isothermal_liquid.isothermal_liquid\"},{\"id\":\"S\",\"label\":\"S\",\"type\":\"input\"}],\"Right\":[{\"id\":\"B\",\"label\":\"B\",\"type\":\"foundation.isothermal_liquid.isothermal_liquid\"},{\"id\":\"F\",\"label\":\"F\",\"type\":\"output\"}],\"Top\":[]}"
  S : PMIOPort  Side=Left
  A : PMIOPort  Port=2  Side=Left
  B : PMIOPort  Port=3  Side=Right
  connections:
  Motion Sensor/RConn3 -- Orifice/LConn1 -- Spool Orifice Hydraulic Force/LConn2
  Hydraulic Force/LConn1 -- Motion Sensor/LConn1 -- S/RConn1
  Orifice/RConn1 -- Spool Orifice Hydraulic Force/LConn1
  Orifice/LConn2 -- A/RConn1
  MTRef Force/LConn1 -- Hydraulic Force/RConn2
  MTRef Sensor/LConn1 -- Motion Sensor/RConn1
  Spool Orifice Hydraulic Force/RConn2 -- Hydraulic Force/RConn1
  Spool Orifice Hydraulic Force/RConn1 -- B/RConn1

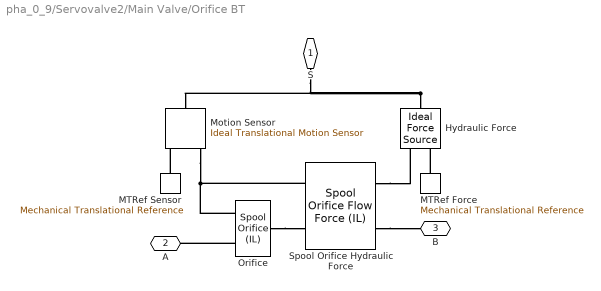
== system pha_0_9/Servovalve2/Main Valve/Orifice BT ==
  Hydraulic Force : fl_lib/Mechanical/Mechanical Sources/Ideal Force Source  Tag=Factory Generic
  MTRef Force : fl_lib/Mechanical/Translational Elements/Mechanical Translational Reference  Tag=Factory Generic
  MTRef Sensor : fl_lib/Mechanical/Translational Elements/Mechanical Translational Reference  Tag=Factory Generic
  Motion Sensor : fl_lib/Mechanical/Mechanical Sensors/Ideal Translational Motion Sensor  Tag=Factory Generic  reference=foundation.enum.MeasurementReference.difference  acceleration_port=false  velocity_port=true  position_port=true  offset=0 m
  Orifice : SimscapeFluids_lib/Isothermal Liquid/Valves & Orifices/Orifices/Spool Orifice (IL)  Tag=Factory Generic  orifice_spec=2  diameter_hole=5e-3 m  num_hole=6  width=24.5 mm  del_S_max=1 m  S_min=-(0.01) mm  open_orientation=1  flow_force_spec=false  clearance=1e-5 m  area_leak=1e-9 m^2  area=inf m^2  Cd=0.7  Re_c=150  smoothing_factor=0  pressure_recovery=false
      settings: InternalSimscapePortConfiguration="{\"Bottom\":[],\"Left\":[{\"id\":\"S\",\"label\":\"S\",\"type\":\"input\"},{\"id\":\"A\",\"label\":\"A\",\"type\":\"foundation.isothermal_liquid.isothermal_liquid\"}],\"Right\":[{\"id\":\"B\",\"label\":\"B\",\"type\":\"foundation.isothermal_liquid.isothermal_liquid\"}],\"Top\":[]}"
  Spool Orifice Hydraulic Force : SimscapeFluids_lib/Isothermal Liquid/Valves & Orifices/Valve Actuators & Forces/Spool Orifice Flow Force (IL)  orifice_spec=2  diameter_hole=0.005 m  num_hole=4  width=24.5 mm  del_S_max=1 m  S_min=-(0.01) mm  open_orientation=1  clearance=0.05 mm  area_leak=(24.5)*(0.05) mm^2  smoothing_factor=0
      settings: LibrarySourceBlock=SimscapeFluids_lib/Isothermal Liquid/Valves & Orifices/Valve Actuators & Forces/Spool Orifice Flow Force (IL)  InternalSimscapePortConfiguration="{\"Bottom\":[],\"Left\":[{\"id\":\"A\",\"label\":\"A\",\"type\":\"foundation.isothermal_liquid.isothermal_liquid\"},{\"id\":\"S\",\"label\":\"S\",\"type\":\"input\"}],\"Right\":[{\"id\":\"B\",\"label\":\"B\",\"type\":\"foundation.isothermal_liquid.isothermal_liquid\"},{\"id\":\"F\",\"label\":\"F\",\"type\":\"output\"}],\"Top\":[]}"
  S : PMIOPort  Side=Left
  A : PMIOPort  Port=2  Side=Left
  B : PMIOPort  Port=3  Side=Right
  connections:
  Motion Sensor/RConn3 -- Orifice/LConn1 -- Spool Orifice Hydraulic Force/LConn2
  Hydraulic Force/LConn1 -- Motion Sensor/LConn1 -- S/RConn1
  MTRef Sensor/LConn1 -- Motion Sensor/RConn1
  Orifice/LConn2 -- A/RConn1
  MTRef Force/LConn1 -- Hydraulic Force/RConn2
  Spool Orifice Hydraulic Force/RConn1 -- B/RConn1
  Spool Orifice Hydraulic Force/RConn2 -- Hydraulic Force/RConn1
  Orifice/RConn1 -- Spool Orifice Hydraulic Force/LConn1

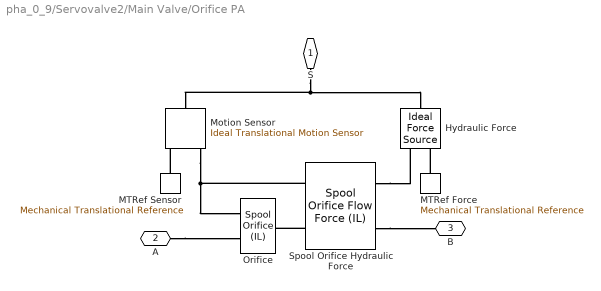
== system pha_0_9/Servovalve2/Main Valve/Orifice PA ==
  Hydraulic Force : fl_lib/Mechanical/Mechanical Sources/Ideal Force Source  Tag=Factory Generic
  MTRef Force : fl_lib/Mechanical/Translational Elements/Mechanical Translational Reference  Tag=Factory Generic
  MTRef Sensor : fl_lib/Mechanical/Translational Elements/Mechanical Translational Reference  Tag=Factory Generic
  Motion Sensor : fl_lib/Mechanical/Mechanical Sensors/Ideal Translational Motion Sensor  Tag=Factory Generic  reference=foundation.enum.MeasurementReference.difference  acceleration_port=false  velocity_port=true  position_port=true  offset=0 m
  Orifice : SimscapeFluids_lib/Isothermal Liquid/Valves & Orifices/Orifices/Spool Orifice (IL)  Tag=Factory Generic  orifice_spec=2  diameter_hole=5e-3 m  num_hole=6  width=24.5 mm  del_S_max=1 m  S_min=-(0.01) mm  open_orientation=1  flow_force_spec=false  clearance=1e-5 m  area_leak=1e-9 m^2  area=inf m^2  Cd=0.7  Re_c=150  smoothing_factor=0  pressure_recovery=false
      settings: InternalSimscapePortConfiguration="{\"Bottom\":[],\"Left\":[{\"id\":\"S\",\"label\":\"S\",\"type\":\"input\"},{\"id\":\"A\",\"label\":\"A\",\"type\":\"foundation.isothermal_liquid.isothermal_liquid\"}],\"Right\":[{\"id\":\"B\",\"label\":\"B\",\"type\":\"foundation.isothermal_liquid.isothermal_liquid\"}],\"Top\":[]}"
  Spool Orifice Hydraulic Force : SimscapeFluids_lib/Isothermal Liquid/Valves & Orifices/Valve Actuators & Forces/Spool Orifice Flow Force (IL)  orifice_spec=2  diameter_hole=0.005 m  num_hole=4  width=24.5 mm  del_S_max=1 m  S_min=-(0.01) mm  open_orientation=1  clearance=0.05 mm  area_leak=(24.5)*(0.05) mm^2  smoothing_factor=0
      settings: LibrarySourceBlock=SimscapeFluids_lib/Isothermal Liquid/Valves & Orifices/Valve Actuators & Forces/Spool Orifice Flow Force (IL)  InternalSimscapePortConfiguration="{\"Bottom\":[],\"Left\":[{\"id\":\"A\",\"label\":\"A\",\"type\":\"foundation.isothermal_liquid.isothermal_liquid\"},{\"id\":\"S\",\"label\":\"S\",\"type\":\"input\"}],\"Right\":[{\"id\":\"B\",\"label\":\"B\",\"type\":\"foundation.isothermal_liquid.isothermal_liquid\"},{\"id\":\"F\",\"label\":\"F\",\"type\":\"output\"}],\"Top\":[]}"
  S : PMIOPort  Side=Left
  A : PMIOPort  Port=2  Side=Left
  B : PMIOPort  Port=3  Side=Right
  connections:
  Spool Orifice Hydraulic Force/RConn2 -- Hydraulic Force/RConn1
  Spool Orifice Hydraulic Force/LConn1 -- Orifice/RConn1
  A/RConn1 -- Orifice/LConn2
  Spool Orifice Hydraulic Force/RConn1 -- B/RConn1
  Spool Orifice Hydraulic Force/LConn2 -- Motion Sensor/RConn3 -- Orifice/LConn1
  MTRef Sensor/LConn1 -- Motion Sensor/RConn1
  MTRef Force/LConn1 -- Hydraulic Force/RConn2
  S/RConn1 -- Motion Sensor/LConn1 -- Hydraulic Force/LConn1

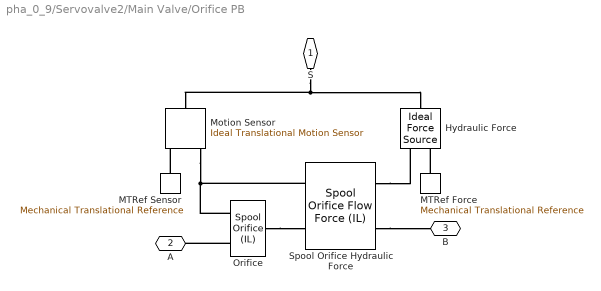
== system pha_0_9/Servovalve2/Main Valve/Orifice PB ==
  Hydraulic Force : fl_lib/Mechanical/Mechanical Sources/Ideal Force Source  Tag=Factory Generic
  MTRef Force : fl_lib/Mechanical/Translational Elements/Mechanical Translational Reference  Tag=Factory Generic
  MTRef Sensor : fl_lib/Mechanical/Translational Elements/Mechanical Translational Reference  Tag=Factory Generic
  Motion Sensor : fl_lib/Mechanical/Mechanical Sensors/Ideal Translational Motion Sensor  Tag=Factory Generic  reference=foundation.enum.MeasurementReference.difference  acceleration_port=false  velocity_port=true  position_port=true  offset=0 m
  Orifice : SimscapeFluids_lib/Isothermal Liquid/Valves & Orifices/Orifices/Spool Orifice (IL)  Tag=Factory Generic  orifice_spec=2  diameter_hole=5e-3 m  num_hole=6  width=24.5 mm  del_S_max=1 m  S_min=0.01 mm  open_orientation=-1  flow_force_spec=false  clearance=1e-5 m  area_leak=1e-9 m^2  area=inf m^2  Cd=0.7  Re_c=150  smoothing_factor=0  pressure_recovery=false
      settings: InternalSimscapePortConfiguration="{\"Bottom\":[],\"Left\":[{\"id\":\"S\",\"label\":\"S\",\"type\":\"input\"},{\"id\":\"A\",\"label\":\"A\",\"type\":\"foundation.isothermal_liquid.isothermal_liquid\"}],\"Right\":[{\"id\":\"B\",\"label\":\"B\",\"type\":\"foundation.isothermal_liquid.isothermal_liquid\"}],\"Top\":[]}"
  Spool Orifice Hydraulic Force : SimscapeFluids_lib/Isothermal Liquid/Valves & Orifices/Valve Actuators & Forces/Spool Orifice Flow Force (IL)  orifice_spec=2  diameter_hole=0.005 m  num_hole=4  width=24.5 mm  del_S_max=1 m  S_min=0.01 mm  open_orientation=-1  clearance=0.05 mm  area_leak=(24.5)*(0.05) mm^2  smoothing_factor=0
      settings: LibrarySourceBlock=SimscapeFluids_lib/Isothermal Liquid/Valves & Orifices/Valve Actuators & Forces/Spool Orifice Flow Force (IL)  InternalSimscapePortConfiguration="{\"Bottom\":[],\"Left\":[{\"id\":\"A\",\"label\":\"A\",\"type\":\"foundation.isothermal_liquid.isothermal_liquid\"},{\"id\":\"S\",\"label\":\"S\",\"type\":\"input\"}],\"Right\":[{\"id\":\"B\",\"label\":\"B\",\"type\":\"foundation.isothermal_liquid.isothermal_liquid\"},{\"id\":\"F\",\"label\":\"F\",\"type\":\"output\"}],\"Top\":[]}"
  S : PMIOPort  Side=Left
  A : PMIOPort  Port=2  Side=Left
  B : PMIOPort  Port=3  Side=Right
  connections:
  Motion Sensor/RConn3 -- Orifice/LConn1 -- Spool Orifice Hydraulic Force/LConn2
  S/RConn1 -- Motion Sensor/LConn1 -- Hydraulic Force/LConn1
  Spool Orifice Hydraulic Force/RConn2 -- Hydraulic Force/RConn1
  Orifice/LConn2 -- A/RConn1
  MTRef Force/LConn1 -- Hydraulic Force/RConn2
  MTRef Sensor/LConn1 -- Motion Sensor/RConn1
  Orifice/RConn1 -- Spool Orifice Hydraulic Force/LConn1
  Spool Orifice Hydraulic Force/RConn1 -- B/RConn1

== system pha_0_9/Servovalve2/Main Valve/Spool Side A ==
  Spool Side A : fl_lib/Isothermal Liquid/Elements/Translational Mechanical Converter (IL)  Tag=Factory Generic  mech_orientation=1  displacement_spec=foundation.enum.DisplacementSpec.Calculate  x0=0 m  interface_area=78 mm^2  dead_volume=1e-4 m^3  pressure_spec=1  environment_pressure=0.101325 MPa  dynamic_compressibility=0  p0=0 + 101325 Pa
      settings: LibrarySourceBlock=fl_lib/Isothermal Liquid/Elements/Translational Mechanical Converter (IL)  InternalSimscapePortConfiguration="{\"Bottom\":[],\"Left\":[{\"id\":\"A\",\"label\":\"A\",\"type\":\"foundation.isothermal_liquid.isothermal_liquid\"},{\"id\":\"C\",\"label\":\"C\",\"type\":\"foundation.mechanical.translational.translational\"}],\"Right\":[{\"id\":\"R\",\"label\":\"R\",\"type\":\"foundation.mechanical.translational.translational\"}],\"Top\":[]}"
  C : PMIOPort  Side=Left
  R : PMIOPort  Port=2  Side=Right
  A : PMIOPort  Port=3  Side=Left
  connections:
  A/RConn1 -- Spool Side A/LConn1
  C/RConn1 -- Spool Side A/LConn2
  Spool Side A/RConn1 -- R/RConn1

== system pha_0_9/Servovalve2/Main Valve/Spool Side B ==
  Spool Side B : fl_lib/Isothermal Liquid/Elements/Translational Mechanical Converter (IL)  Tag=Factory Generic  mech_orientation=-1  displacement_spec=foundation.enum.DisplacementSpec.Calculate  x0=-(0) m  interface_area=78 mm^2  dead_volume=1e-4 m^3  pressure_spec=1  environment_pressure=0.101325 MPa  dynamic_compressibility=0  p0=0 + 101325 Pa
      settings: LibrarySourceBlock=fl_lib/Isothermal Liquid/Elements/Translational Mechanical Converter (IL)  InternalSimscapePortConfiguration="{\"Bottom\":[],\"Left\":[{\"id\":\"A\",\"label\":\"A\",\"type\":\"foundation.isothermal_liquid.isothermal_liquid\"},{\"id\":\"C\",\"label\":\"C\",\"type\":\"foundation.mechanical.translational.translational\"}],\"Right\":[{\"id\":\"R\",\"label\":\"R\",\"type\":\"foundation.mechanical.translational.translational\"}],\"Top\":[]}"
  C : PMIOPort  Side=Left
  R : PMIOPort  Port=2  Side=Right
  A : PMIOPort  Port=3  Side=Left
  connections:
  R/RConn1 -- Spool Side B/RConn1
  Spool Side B/LConn1 -- A/RConn1
  Spool Side B/LConn2 -- C/RConn1

== stateflow chart pha_0_9/Chart2 ==
  state pritisak_veci_od_1_5
    entry:
    y1 = 2;
    y2 = -1;
    during:
    y1 = 2;
    y2 = -1
  state pritisak_manji_od_1_4
    entry:
    y1 = 2;
    y2 = 1;
    during:
    y1 = 2;
    y2 = 1
  (default) -> pritisak_veci_od_1_5
  pritisak_veci_od_1_5 -> pritisak_manji_od_1_4 : [x<1.5]
  pritisak_manji_od_1_4 -> pritisak_veci_od_1_5 : [x > 1.4]
  data: x input; y1 output; y2 output
